simulink library "create_index_vector_lib"  (R2020b)
settings: Solver=VariableStepAuto  StartTime=0.0  StopTime=10.0  RelTol=1e-3
settings Model: Creator=rsub  LastModifiedBy=rsub

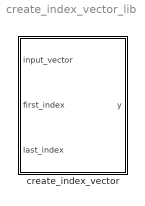
== system create_index_vector_lib ==
  create_index_vector : Subsystem

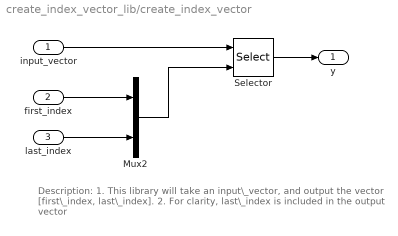
== system create_index_vector_lib/create_index_vector ==
  note: Description:
      | 1. This library will take an input\_vector, and output the vector [first\_index, last\_index].
      | 2. For clarity, last\_index is included in the output vector
  input_vector : Inport
  first_index : Inport  Port=2
  last_index : Inport  Port=3
  Mux2 : Mux  Inputs=2
  Selector : Selector  IndexMode=Zero-based  InputPortWidth=6  IndexOptions=Starting and ending indices (port)  Indices=[1 3]  OutputSizes=1
      settings: AttributesFormatString=%<IndexOptions>
  y : Outport
  wires:
  last_index/1 -> Mux2/2
  Mux2/1 -> Selector/2
  first_index/1 -> Mux2/1
  Selector/1 -> y/1
  input_vector/1 -> Selector/1
